simulink model "M_DYN"  (R2022a)
settings: Solver=ode4  StartTime=0.0  StopTime=0.04  FixedStep=0.01  RelTol=1e-3
PreLoadFcn:
  | listing = dir;
  | if (contains([listing .name], 'FLCC')) && (contains([listing .name], 'DYN'))
  |     addpath('./DYN', './FLCC');
  | elseif (contains([listing .name], 'M_DYN.slx'))
  |     addpath('../DYN', '../FLCC');
  | else
  | 
  | end
  | 
  | load('f16data.mat');
  | load('BUS_STRUCTURE_DYN.mat');
  | load('BUS_STRUCTURE_FLCC.mat');
InitFcn:
  | listing = dir;
  | if (contains([listing .name], 'FLCC')) && (contains([listing .name], 'DYN'))
  |     addpath('./DYN', './FLCC');
  | elseif (contains([listing .name], 'M_DYN.slx'))
  |     addpath('../DYN', '../FLCC');
  | else
  | 
  | end
  | 
  | load('f16data.mat');
  | load('BUS_STRUCTURE_DYN.mat');
  | load('BUS_STRUCTURE_FLCC.mat');
values from neighbouring files (symbols this model uses):
  f16data =     [f16data.mat]
libraries: simulink_extras x6, aerolibatmos2 x1
settings Model: Creator=ASCL  LastModifiedBy=ASCL
settings DataIOCC: SaveOutput=off  SignalLogging=off  DSMLogging=off  SaveTime=off  ReturnWorkspaceOutputs=off
settings OptimizationCC: BlockReduction=off  DefaultParameterBehavior=Inlined  UseDivisionForNetSlopeComputation=on  GainParamInheritBuiltInType=on  UseFloatMulNetSlope=on  ExpressionFolding=off  PassReuseOutputArgsAs=Individual arguments  ZeroExternalMemoryAtStartup=off  ZeroInternalMemoryAtStartup=off  EfficientFloat2IntCast=on  LifeSpan=inf  OptimizeBlockOrder=speed  DifferentSizesBufferReuse=on  EfficientTunableParamExpr=on
settings DebuggingCC: SignalInfNanChecking=warning  ReadBeforeWriteMsg=EnableAllAsError  WriteAfterWriteMsg=EnableAllAsError  WriteAfterReadMsg=EnableAllAsError  IntegerOverflowMsg=error  ParameterTunabilityLossMsg=error  UniqueDataStoreMsg=error  AssertControl=DisableAll  NonBusSignalsTreatedAsBus=error  SFInvalidInputDataAccessInChartInitDiag=error  SFTransitionOutsideNaturalParentDiag=error  SFUnreachableExecutionPathDiag=error  SFUndirectedBroadcastEventsDiag=error  IntegerSaturationMsg=error
settings HardwareCC: ProdBitPerPointer=32  ProdBitPerSizeT=32  ProdBitPerPtrDiffT=32  ProdLargestAtomicInteger=Long  ProdLargestAtomicFloat=Double  ProdEndianess=BigEndian  ProdWordSize=32  ProdLongLongMode=on  ProdHWDeviceType=Freescale->MPC83xx
settings ModelReferenceCC: ModelReferenceNumInstancesAllowed=Single
settings SFSimCC: CompileTimeRecursionLimit=0  EnableRuntimeRecursion=off  MATLABDynamicMemAlloc=off
settings RTWCC: SystemTargetFile=ert.tlc  TemplateMakefile=ert_default_tmf  GenerateReport=on  RTWUseSimCustomCode=on  BuildConfiguration=Faster Runs  IncludeHyperlinkInReport=on  LaunchReport=on  GenerateTraceInfo=on  GenerateTraceReport=on  GenerateTraceReportSl=on  GenerateTraceReportSf=on  GenerateTraceReportEml=on
settings CodeAppCC: ForceParamTrailComments=on  IgnoreCustomStorageClasses=off  OperatorAnnotations=on  SimulinkDataObjDesc=on  SFDataObjDesc=on  MATLABFcnDesc=on  InsertBlockDesc=on  StateflowObjectComments=on  MATLABSourceComments=on  EnableCustomComments=on  InlinedPrmAccess=Macros  ReqsInCode=on
settings ERTTargetCC: TargetLangStandard=C99 (ISO)  UtilityFuncGeneration=Shared location  GenerateSampleERTMain=on  IncludeMdlTerminateFcn=off  CombineSignalStateStructs=on  SupportAbsoluteTime=off  SupportNonFinite=off  SupportVariableSizeSignals=on  ParenthesesLevel=Standards  CastingMode=Standards  GenerateSharedConstants=off  InlinedParameterPlacement=NonHierarchical  ERTCustomFileTemplate=example_file_process.tlc  RateTransitionBlockCode=Function  PreserveIfCondition=on  ConvertIfToSwitch=off  EnableSignedLeftShifts=off  EnableSignedRightShifts=off

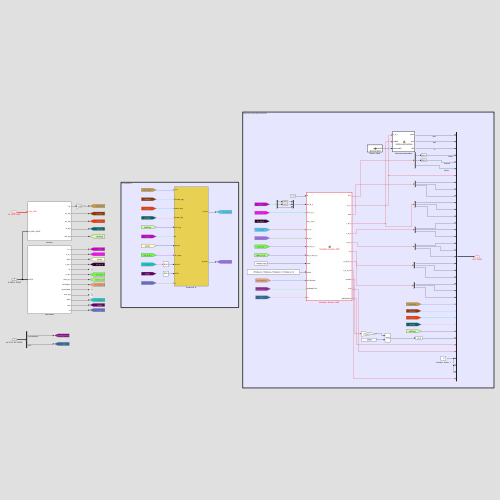
[thumbnail: Simulink's stored preview of the top-level diagram]
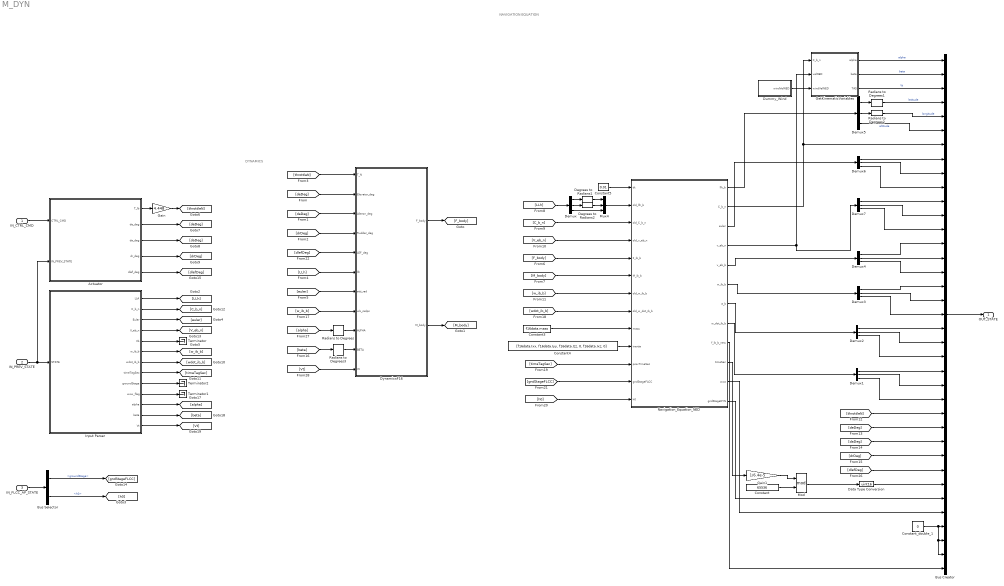
== system M_DYN ==
  note: DYNAMICS
  note: NAVIGATION EQUATION
  IN_CTRL_CMD : Inport  OutDataTypeStr=Bus: BUS_FLCC_CTRL_CMD  Interpolate=off  BusOutputAsStruct=on
  IN_PREV_STATE : Inport  Port=2  OutDataTypeStr=Bus: BUS_DYN_STATE  Interpolate=off  BusOutputAsStruct=on
  IN_FLCC_AP_STATE : Inport  Port=3  OutDataTypeStr=Bus: BUS_FLCC_AP_STATE  BusOutputAsStruct=on
  Actuator : Subsystem
  Bus Creator : BusCreator  Inputs=37  OutDataTypeStr=Bus: BUS_DYN_STATE  NonVirtualBus=on
      settings: InheritFromInputs=off
  Bus Selector : BusSelector  OutputSignals=groundStage,h0
  Constant : Constant  Value=65536
  Constant3 : Constant  Value=f16data.mass
  Constant4 : Constant  Value=[f16data.Ixx, f16data.Iyy, f16data.Izz, 0, f16data.Ixz, 0]
  Constant5 : Constant  Value=0.01
  Constant_double_1 : Constant  Value=0  OutDataTypeStr=double
  Data Type Conversion : DataTypeConversion  OutDataTypeStr=uint16  RndMeth=Round  SaturateOnIntegerOverflow=off
  Degrees to Radians1 : simulink_extras/Transformations/Degrees to Radians
  Degrees to Radians2 : simulink_extras/Transformations/Degrees to Radians
  Demux{,1..7} (8 alike) : Demux  Outputs=3
  Dummy_Wind : MATLAB Function  TreatAsAtomicUnit=on
  DynamicsF16 : Subsystem
  Gain : Gain  Gain=4.448
  Gain1 : Gain  Gain=1/6.4e-5
  GetKinematicVariables : MATLAB Function  TreatAsAtomicUnit=on
  Input Parser : Subsystem
  Mod : Math  Operator=mod  OutputSignalType=real
  Mux4 : Mux  Inputs=3
  Navigation_Equation_NED : MATLAB Function  TreatAsAtomicUnit=on
  Radians to Degrees{,1..3} (4 alike) : simulink_extras/Transformations/Radians to Degrees
  Terminator : Terminator
  Terminator1 : Terminator
  Terminator2 : Terminator
  OUT_STATE : Outport  OutDataTypeStr=Bus: BUS_DYN_STATE  VectorParamsAs1DForOutWhenUnconnected=off  BusOutputAsStruct=on
  wires:
  Actuator/4(dr_deg) -> [drDeg]
  Demux/2 -> Degrees to Radians2/1
  Demux6/3 -> Bus Creator/10
  Navigation_Equation_NED/2(C_b_n) -> Bus Creator/7, GetKinematicVariables/1(C_b_n)
  Navigation_Equation_NED/10(timeSec) -> Gain1/1
  Data Type Conversion/1 -> Bus Creator/31
  [deDeg] -> DynamicsF16/2(Elevator_deg)
  Navigation_Equation_NED/3(euler) -> Demux6/1
  [timeTagSec] -> Navigation_Equation_NED/11(prevTimeSec)
  Demux1/3 -> Bus Creator/25
  Demux1/2 -> Bus Creator/24
  [F_body] -> Navigation_Equation_NED/5(F_ib_b)
  Demux6/1 -> Bus Creator/8
  Demux3/3 -> Bus Creator/19
  Navigation_Equation_NED/7(a_b) -> Demux2/1
  Demux/3 -> Mux4/3
  Navigation_Equation_NED/5(v_eb_b) -> Demux4/1
  Mux4/1 -> Navigation_Equation_NED/2(old_llh_b)
  Demux3/1 -> Bus Creator/17
  [C_b_n] -> Navigation_Equation_NED/3(old_C_b_n)
  Demux4/2 -> Bus Creator/15
  [w_ib_b] -> DynamicsF16/8(wb_radps)
  [drDeg] -> DynamicsF16/4(Rudder_deg)
  Demux1/1 -> Bus Creator/23
  [euler] -> DynamicsF16/7(atti_rad)
  Demux4/3 -> Bus Creator/16
  [daDeg] -> Bus Creator/28
  Demux3/2 -> Bus Creator/18
  Degrees to Radians2/1 -> Mux4/2
  [wdot_ib_b] -> Navigation_Equation_NED/8(old_w_dot_ib_b)
  Actuator/1(T_lb) -> Gain/1
  Input Parser/3(Euler) -> [euler]
  Actuator/3(da_deg) -> [daDeg]
  Radians to Degrees2/1 -> Bus Creator/5  "longitude"
  Demux4/1 -> Bus Creator/14
  Input Parser/1(LLA) -> [LLh]
  IN_CTRL_CMD/1 -> Actuator/1(CTRL_CMD)
  Actuator/2(de_deg) -> [deDeg]
  [daDeg] -> DynamicsF16/3(Aileron_deg)
  Demux6/2 -> Bus Creator/9
  [V_eb_n] -> Navigation_Equation_NED/4(old_v_eb_n)
  [deDeg] -> Bus Creator/27
  Navigation_Equation_NED/1(llh_b) -> Demux5/1
  Demux2/2 -> Bus Creator/21
  Degrees to Radians1/1 -> Mux4/1
  Input Parser/6(w_ib_b) -> [w_ib_b]
  Demux2/3 -> Bus Creator/22
  DynamicsF16/1(F_body) -> [F_body]
  Constant5/1 -> Navigation_Equation_NED/1(dt)
  Bus Creator/1 -> OUT_STATE/1
  Demux5/2 -> Radians to Degrees2/1
  [w_ib_b] -> Navigation_Equation_NED/7(old_w_ib_b)
  Input Parser/7(wdot_ib_b) -> [wdot_ib_b]
  Input Parser/8(timeTagSec) -> [timeTagSec]
  Navigation_Equation_NED/8(w_dot_ib_b) -> Demux1/1
  [LLh] -> DynamicsF16/6(llh)
  Radians to Degrees1/1 -> Bus Creator/4  "latitude"
  [throttleN] -> DynamicsF16/1(T_N)
  Demux5/1 -> Radians to Degrees1/1
  Demux5/3 -> Bus Creator/6  "altitude"
  Gain/1 -> [throttleN]
  [LLh] -> Demux/1
  Demux/1 -> Degrees to Radians1/1
  DynamicsF16/2(M_body) -> [M_body]
  Navigation_Equation_NED/4(v_eb_n) -> Demux7/1, GetKinematicVariables/2(velNED)
  Constant4/1 -> Navigation_Equation_NED/10(inertia)
  Constant3/1 -> Navigation_Equation_NED/9(mass)
  [drDeg] -> Bus Creator/29
  Demux2/1 -> Bus Creator/20
  [throttleN] -> Bus Creator/26
  IN_PREV_STATE/1 -> Actuator/2(IN_PREV_STATE), Input Parser/1(STATE)
  [M_body] -> Navigation_Equation_NED/6(M_ib_b)
  Gain1/1 -> Mod/1
  Mod/1 -> Data Type Conversion/1
  Constant/1 -> Mod/2
  Demux7/2 -> Bus Creator/12
  Demux7/1 -> Bus Creator/11
  Demux7/3 -> Bus Creator/13
  Input Parser/4(V_eb_n) -> [V_eb_n]
  Input Parser/2(C_b_n) -> [C_b_n]
  Input Parser/9(groundStage) -> Terminator2/1
  [gndStageFLCC] -> Navigation_Equation_NED/12(gndStageFLCC)
  Navigation_Equation_NED/11(wow) -> Bus Creator/33
  Actuator/5(dlef_deg) -> [dlefDeg]
  [dlefDeg] -> DynamicsF16/5(LEF_deg)
  Dummy_Wind/1(windVelNED) -> GetKinematicVariables/3(windVelNED)
  GetKinematicVariables/1(alpha) -> Bus Creator/1  "alpha"
  GetKinematicVariables/2(beta) -> Bus Creator/2  "beta"
  GetKinematicVariables/3(TAS) -> Bus Creator/3  "Vt"
  [dlefDeg] -> Bus Creator/30
  Constant_double_1/1 -> Bus Creator/34, Bus Creator/36, Bus Creator/35
  Input Parser/11(alpha) -> [alpha]
  Input Parser/12(beta) -> [beta]
  Input Parser/13(Vt) -> [Vt]
  [alpha] -> Radians to Degrees/1
  [beta] -> Radians to Degrees3/1
  [Vt] -> DynamicsF16/11(Vt)
  Radians to Degrees/1 -> DynamicsF16/9(ALPHA)
  Radians to Degrees3/1 -> DynamicsF16/10(BETA)
  Navigation_Equation_NED/12(gndStageDYN) -> Bus Creator/32
  Navigation_Equation_NED/6(w_ib_b) -> Demux3/1
  Navigation_Equation_NED/9(f_ib_b_new) -> Bus Creator/37
  Input Parser/5(Vb) -> Terminator/1
  Input Parser/10(wow_flag) -> Terminator1/1
  IN_FLCC_AP_STATE/1 -> Bus Selector/1
  Bus Selector/1 -> [gndStageFLCC]  "<groundStage>"
  Bus Selector/2 -> [h0]  "<h0>"
  [h0] -> Navigation_Equation_NED/13(h0)

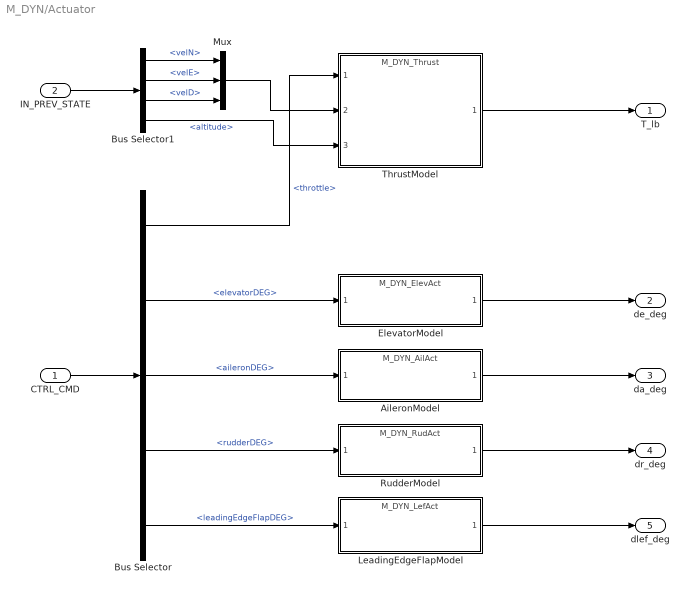
== system M_DYN/Actuator ==
  CTRL_CMD : Inport  OutDataTypeStr=Bus: BUS_FLCC_CTRL_CMD  BusOutputAsStruct=on
  IN_PREV_STATE : Inport  Port=2
  AileronModel : ModelReference  ModelNameDialog=M_DYN_AilAct.slx  ModelReferenceVersion=1.69
  Bus Selector : BusSelector  OutputSignals=throttle,elevatorDEG,aileronDEG,rudderDEG,leadingEdgeFlapDEG
  Bus Selector1 : BusSelector  OutputSignals=velN,velE,velD,altitude
  ElevatorModel : ModelReference  ModelNameDialog=M_DYN_ElevAct.slx  ModelReferenceVersion=1.68
  LeadingEdgeFlapModel : ModelReference  ModelNameDialog=M_DYN_LefAct.slx  SimulationMode=Normal  ModelReferenceVersion=1.75
  Mux : Mux  Inputs=3
  RudderModel : ModelReference  ModelNameDialog=M_DYN_RudAct.slx  ModelReferenceVersion=1.70
  ThrustModel : ModelReference  ModelNameDialog=M_DYN_Thrust.slx  ModelReferenceVersion=1.128
  T_lb : Outport
  de_deg : Outport  Port=2
  da_deg : Outport  Port=3
  dr_deg : Outport  Port=4
  dlef_deg : Outport  Port=5
  wires:
  Bus Selector/1 -> ThrustModel/1  "<throttle>"
  Bus Selector/3 -> AileronModel/1  "<aileronDEG>"
  Bus Selector/2 -> ElevatorModel/1  "<elevatorDEG>"
  Bus Selector/4 -> RudderModel/1  "<rudderDEG>"
  CTRL_CMD/1 -> Bus Selector/1
  ThrustModel/1 -> T_lb/1
  ElevatorModel/1 -> de_deg/1
  RudderModel/1 -> dr_deg/1
  AileronModel/1 -> da_deg/1
  IN_PREV_STATE/1 -> Bus Selector1/1
  Bus Selector1/1 -> Mux/1  "<velN>"
  Bus Selector1/2 -> Mux/2  "<velE>"
  Bus Selector1/3 -> Mux/3  "<velD>"
  Bus Selector1/4 -> ThrustModel/3  "<altitude>"
  Mux/1 -> ThrustModel/2
  LeadingEdgeFlapModel/1 -> dlef_deg/1
  Bus Selector/5 -> LeadingEdgeFlapModel/1  "<leadingEdgeFlapDEG>"

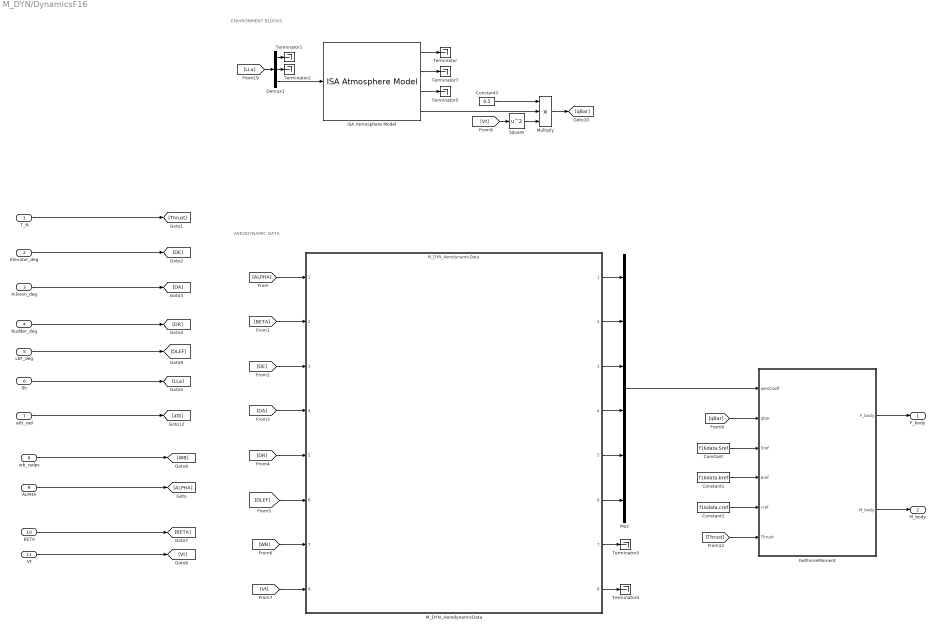
== system M_DYN/DynamicsF16 ==
  note: AERODYNAMIC DATA
  note: ENVIRONMENT BLOCKS
  T_N : Inport
  Elevator_deg : Inport  Port=2
  Aileron_deg : Inport  Port=3
  Rudder_deg : Inport  Port=4
  LEF_deg : Inport  Port=5
  llh : Inport  Port=6
  atti_rad : Inport  Port=7
  wb_radps : Inport  Port=8
  ALPHA : Inport  Port=9
  BETA : Inport  Port=10
  Vt : Inport  Port=11
  Constant : Constant  Value=f16data.Sref
  Constant1 : Constant  Value=f16data.bref
  Constant2 : Constant  Value=f16data.cref
  Constant3 : Constant  Value=0.5
  Demux1 : Demux  Outputs=3
  GetForceMoment : MATLAB Function  TreatAsAtomicUnit=on
  ISA Atmosphere Model : aerolibatmos2/ISA Atmosphere Model  custom=off  g=9.80665  gamma=1.4  R=287.0531  L=0.0065  h_trop=11000  h_strat=20000  rho0=1.225  P0=101325  T0=288.15  h0=0
  M_DYN_AerodynamicData : ModelReference  ModelNameDialog=M_DYN_AerodynamicData.slx  SimulationMode=Normal  ModelReferenceVersion=1.96
  Multiply : Product  Inputs=3
  Mux : Mux  Inputs=6
  Square : Math  Operator=square  SignedPower=on
  Terminator{,1..5,7} (7 alike) : Terminator
  F_body : Outport  VectorParamsAs1DForOutWhenUnconnected=off
  M_body : Outport  Port=2  VectorParamsAs1DForOutWhenUnconnected=off
  wires:
  ISA Atmosphere Model/4 -> Multiply/2
  ISA Atmosphere Model/1 -> Terminator/1
  ISA Atmosphere Model/3 -> Terminator5/1
  T_N/1 -> [Thrust]
  Elevator_deg/1 -> [DE]
  Aileron_deg/1 -> [DA]
  Rudder_deg/1 -> [DR]
  atti_rad/1 -> [atti]
  llh/1 -> [LLa]
  [LLa] -> Demux1/1
  Demux1/3 -> ISA Atmosphere Model/1
  Demux1/1 -> Terminator1/1
  Demux1/2 -> Terminator2/1
  LEF_deg/1 -> [DLEF]
  [ALPHA] -> M_DYN_AerodynamicData/1
  [BETA] -> M_DYN_AerodynamicData/2
  [DE] -> M_DYN_AerodynamicData/3
  [DA] -> M_DYN_AerodynamicData/4
  [DR] -> M_DYN_AerodynamicData/5
  [DLEF] -> M_DYN_AerodynamicData/6
  [WB] -> M_DYN_AerodynamicData/7
  wb_radps/1 -> [WB]
  [Vt] -> M_DYN_AerodynamicData/8
  M_DYN_AerodynamicData/1 -> Mux/1
  M_DYN_AerodynamicData/2 -> Mux/2
  M_DYN_AerodynamicData/3 -> Mux/3
  M_DYN_AerodynamicData/4 -> Mux/4
  M_DYN_AerodynamicData/5 -> Mux/5
  M_DYN_AerodynamicData/6 -> Mux/6
  Mux/1 -> GetForceMoment/1(aeroCoeff)
  GetForceMoment/1(F_body) -> F_body/1
  GetForceMoment/2(M_body) -> M_body/1
  [qBar] -> GetForceMoment/2(qbar)
  Constant/1 -> GetForceMoment/3(Sref)
  Constant2/1 -> GetForceMoment/5(cref)
  Constant1/1 -> GetForceMoment/4(bref)
  [Thrust] -> GetForceMoment/6(Thrust)
  ISA Atmosphere Model/2 -> Terminator7/1
  [Vt] -> Square/1
  Square/1 -> Multiply/3
  Constant3/1 -> Multiply/1
  Multiply/1 -> [qBar]
  M_DYN_AerodynamicData/8 -> Terminator4/1
  M_DYN_AerodynamicData/7 -> Terminator3/1
  ALPHA/1 -> [ALPHA]
  BETA/1 -> [BETA]
  Vt/1 -> [Vt]

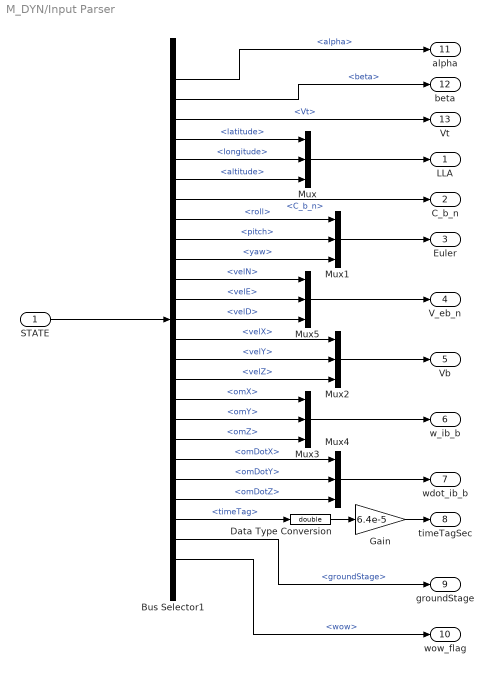
== system M_DYN/Input Parser ==
  STATE : Inport  OutDataTypeStr=Bus: BUS_DYN_STATE
  Bus Selector1 : BusSelector  OutputSignals=alpha,beta,Vt,latitude,longitude,altitude,C_b_n,roll,pitch,yaw,velN,velE,velD,velX,velY,velZ,omX,omY,omZ,omDotX,omDotY,omDotZ,timeTag,groundStage,wow
  Data Type Conversion : DataTypeConversion  OutDataTypeStr=double  SaturateOnIntegerOverflow=off  RndMeth=Floor
  Gain : Gain  Gain=6.4e-5
  Mux{,1..5} (6 alike) : Mux  Inputs=3
  LLA : Outport
  C_b_n : Outport  Port=2
  Euler : Outport  Port=3
  V_eb_n : Outport  Port=4
  Vb : Outport  Port=5
  w_ib_b : Outport  Port=6
  wdot_ib_b : Outport  Port=7
  timeTagSec : Outport  Port=8
  groundStage : Outport  Port=9
  wow_flag : Outport  Port=10
  alpha : Outport  Port=11
  beta : Outport  Port=12
  Vt : Outport  Port=13
  wires:
  Bus Selector1/5 -> Mux/2  "<longitude>"
  Bus Selector1/4 -> Mux/1  "<latitude>"
  Bus Selector1/6 -> Mux/3  "<altitude>"
  Mux3/1 -> w_ib_b/1
  Mux/1 -> LLA/1
  STATE/1 -> Bus Selector1/1
  Bus Selector1/18 -> Mux3/2  "<omY>"
  Bus Selector1/19 -> Mux3/3  "<omZ>"
  Bus Selector1/17 -> Mux3/1  "<omX>"
  Bus Selector1/16 -> Mux2/3  "<velZ>"
  Bus Selector1/15 -> Mux2/2  "<velY>"
  Bus Selector1/14 -> Mux2/1  "<velX>"
  Bus Selector1/10 -> Mux1/3  "<yaw>"
  Bus Selector1/9 -> Mux1/2  "<pitch>"
  Bus Selector1/8 -> Mux1/1  "<roll>"
  Mux1/1 -> Euler/1
  Mux2/1 -> Vb/1
  Bus Selector1/21 -> Mux4/2  "<omDotY>"
  Bus Selector1/20 -> Mux4/1  "<omDotX>"
  Bus Selector1/22 -> Mux4/3  "<omDotZ>"
  Mux4/1 -> wdot_ib_b/1
  Bus Selector1/23 -> Data Type Conversion/1  "<timeTag>"
  Data Type Conversion/1 -> Gain/1
  Gain/1 -> timeTagSec/1
  Bus Selector1/7 -> C_b_n/1  "<C_b_n>"
  Bus Selector1/12 -> Mux5/2  "<velE>"
  Bus Selector1/11 -> Mux5/1  "<velN>"
  Bus Selector1/13 -> Mux5/3  "<velD>"
  Mux5/1 -> V_eb_n/1
  Bus Selector1/24 -> groundStage/1  "<groundStage>"
  Bus Selector1/25 -> wow_flag/1  "<wow>"
  Bus Selector1/1 -> alpha/1  "<alpha>"
  Bus Selector1/2 -> beta/1  "<beta>"
  Bus Selector1/3 -> Vt/1  "<Vt>"

== matlab function M_DYN/Dummy_Wind ==
  data: windVelNED output
function windVelNED = Dummy_Wind()
windVelNED = zeros(3,1);

== matlab function M_DYN/DynamicsF16/GetForceMoment ==
  data: F_body output; M_body output; aeroCoeff input; qbar input; Sref input; bref input; cref input; Thrust input
function [F_body, M_body] = GetForceMoment(aeroCoeff, qbar, Sref, bref, cref, Thrust)

F_body = zeros(3,1);
M_body = zeros(3,1);

% Force [N]
F_body(1) = aeroCoeff(1) * qbar * Sref + Thrust;
F_body(2) = aeroCoeff(2) * qbar * Sref;
F_body(3) = aeroCoeff(3) * qbar * Sref;

% Moment [N-m]
M_body(1) = aeroCoeff(4) * qbar * Sref * bref;
M_body(2) = aeroCoeff(5) * qbar * Sref * cref;
M_body(3) = aeroCoeff(6) * qbar * Sref * bref;

== matlab function M_DYN/Navigation_Equation_NED ==
  data: dt input; llh_b output; old_llh_b input; old_C_b_n input; old_v_eb_n input; F_ib_b input; M_ib_b input; old_w_ib_b input; old_w_dot_ib_b input; mass input; inertia input; C_b_n output; euler output; v_eb_n output; v_eb_b output; w_ib_b output; a_b output; w_dot_ib_b output; f_ib_b_new output; timeSec output; prevTimeSec input; gndStageFLCC input; wow output; h0 input; gndStageDYN output
function [llh_b, C_b_n, euler, v_eb_n, v_eb_b, w_ib_b, a_b, w_dot_ib_b, f_ib_b_new, timeSec, wow, gndStageDYN]   = Navigation_Equation_NED(dt, old_llh_b, old_C_b_n, old_v_eb_n, F_ib_b, M_ib_b, old_w_ib_b, old_w_dot_ib_b, mass, inertia, prevTimeSec, gndStageFLCC, h0)
% Reference:    Groves, Paul D. "Principles of GNSS, inertial, and 
%               multisensor integrated navigation systems, [Book review]."
%               IEEE Aerospace and Electronic Systems Magazine 30.2 (2015): 26-27.
%
% INPUTS:
%   dt          time interval between updates [s]
%   old_llh_b   previous latitude, longitude, height [rad, rad, m]
%   old_C_b_n   previous body-to-NED coordinate transformation matrix
%   old_v_eb_n  previous velocity of body frame w.r.t. ECEF frame,
%               resolved along north, east, and down [m/s]
%   F_ib_b      (non-gravitational) force of body frame w.r.t.
%               ECEF frame, resolved along body-frame axes, averaged over
%               time interval [m/s^2]
%   M_ib_b      net moment of body frame w.r.t. ECI frame, 
%               resolved about body-frame axes [kg m^2 rad/s]
%   old_w_ib_b  previous body angular rate w.r.t. ECI frame,
%               resolved about body axes [rad/s]
%   old_w_dot_ib_b
%               previous time rate of body angular rate w.r.t. ECI frame,
%               resolved about body axes [rad/s^2]
%   mass        [kg]
%   inertia     [kg m^2]
%   prevTimeSec [sec]
%   prevFlightStage uint8 flag
%
% OUTPUTS: 
%   llh_b       latitude, longitude, height [rad, rad, m]
%   C_b_n       body-to-NED coordinate transformation matrix
%   v_eb_n      velocity of body frame w.r.t. ECEF frame,
%               resolved along north, east, and down [m/s]
%   w_ib_b      body angular rate [rad/s]
%   w_dot_ib_b  time rate of body angular rate [rad/s^2]
%   a_b         body acceleration [m/s^2]
%   euler       [rad]
%   v_eb_b      body velocity [m/s]
%   timeSec     [sec]
%   flightStage uint8
%   wow         boolean

%% [0] Initialize Outputs
llh_b   = zeros(3,1);
C_b_n   = zeros(3,3);
v_eb_n  = zeros(3,1);
w_ib_b  = zeros(3,1);
w_dot_ib_b  = zeros(3,1);
a_b     = zeros(3,1);
euler   = zeros(3,1);
v_eb_b  = zeros(3,1);
f_ib_b_new = zeros(3,1);
timeSec = 0;
wow = true;
gndStageDYN = gndStageFLCC;

if gndStageDYN == uint8(9)
    llh_b = old_llh_b;
    timeSec = prevTimeSec + dt;
    return
else
end

%% [1] Define Constant Parameters
w_ie    = 7.2921159E-5;     % Earth rotation rate [rad/s]
R_0     = 6378137;          % WGS84 Equatorial radius [m]
R_P     = 6356752.31425;    %WGS84 Polar radius [m]
e       = 0.0818191908425;  % WGS84 eccentricity
f       = 1 / 298.257223563;%WGS84 flattening
mu      = 3.986004418E14;   %WGS84 Earth gravitational constant [m^3 s^-2]

Ib      = [inertia(1), -inertia(4), -inertia(5);...
          -inertia(4),  inertia(2), -inertia(6);...
          -inertia(5), -inertia(6),  inertia(3)];
%                           % Moment of inertia [kg m^2]

% Tolerance for compared to zero operation
TOL     = eps(0.5);

%% [2] ATTITUDE UPDATE

% Calculate w_ib_b: angular rate of body frame w.r.t. ECI frame,
%           resolved about body axes, averaged over time interval [rad/s]
w_dot_ib_b  = Ib\(M_ib_b - cross(old_w_ib_b, Ib*old_w_ib_b));
% w_ib_b      = old_w_ib_b + 0.5 * dt * (w_dot_ib_b + old_w_dot_ib_b); 
w_ib_b      = old_w_ib_b + dt * w_dot_ib_b;

% START: TRICK for ground motion ------------------------------------------
if gndStageDYN <= uint8(4)
    w_ib_b(1) = 0.0;
    w_ib_b(2) = 0.0;
    w_dot_ib_b = (w_ib_b - old_w_ib_b ) / (0.5*dt) - old_w_dot_ib_b;
end
% END: TRICK for ground motion --------------------------------------------

% First, Calculate attitude increment, magnitude, and skew-symmetric matrix
alpha_ib_b  = w_ib_b * dt;
if abs(alpha_ib_b' * alpha_ib_b - 0) < TOL % (alpha_ib_b' * alpha_ib_b == 0)
    mag_alpha   = 0.0;
else
    mag_alpha   = sqrt(alpha_ib_b' * alpha_ib_b);
end

Alpha_ib_b  = [             0, -alpha_ib_b(3),  alpha_ib_b(2); ...
                alpha_ib_b(3),              0, -alpha_ib_b(1); ...
               -alpha_ib_b(2),  alpha_ib_b(1),             0];

w_ie_n      = w_ie * [cos(old_llh_b(1)); 0; -sin(old_llh_b(1))];

% From (5.44), determine the angular rate of the NED frame
% w.r.t the ECEF frame, resolved about NED
old_N_E     = R_0 * (1-e^2) / sqrt( 1 - (e * sin(old_llh_b(1)))^2 );
old_M_E_norm1 = 1 - (e * sin(old_llh_b(1)))^2;
if (old_M_E_norm1 > 0.000001)
    old_M_E_norm2 = sqrt(old_M_E_norm1);
    old_M_E_norm3 = old_M_E_norm1 * old_M_E_norm2;
    old_M_E = R_0 / old_M_E_norm3;
else
    old_M_E_norm2 = 0.0;
    old_M_E_norm3 = 0.0;
    old_M_E = R_0 / 0.97;
end

old_w_en_n = [old_v_eb_n(2) / (old_N_E + old_llh_b(3));...
             -old_v_eb_n(1) / (old_M_E + old_llh_b(3));...
             -old_v_eb_n(2) * tan(old_llh_b(1)) / (old_N_E + old_llh_b(3))];


%% [3] SPECIFIC FORCE FRAME TRANSFORMATION
% Calculate ave_C_b_e: the average body-to-ECEF-frame transformation matrix
%           over the update interval using (5.84) and (5.85)
temp_w_enie_n   = old_w_en_n + w_ie_n;
skew_w_enie_n   = [               0,-temp_w_enie_n(3), temp_w_enie_n(2);...
                   temp_w_enie_n(3),                0,-temp_w_enie_n(1);...
                  -temp_w_enie_n(2), temp_w_enie_n(1),                0];

if (mag_alpha > 1.E-8)
    ave_C_b_n = old_C_b_n * (eye(3) + (1 - cos(mag_alpha)) / mag_alpha^2 ...
        * Alpha_ib_b + (1 - sin(mag_alpha) / mag_alpha) / mag_alpha^2 ...
        * Alpha_ib_b * Alpha_ib_b) ...
        - 0.5 * skew_w_enie_n * old_C_b_n;
else
     ave_C_b_n = old_C_b_n ...
        - 0.5 * skew_w_enie_n * old_C_b_n;
end %if mag_alpha     

% Orthonormalize DCM
ave_C_b_n   = quat2rotm(quatnormalize(rotm2quat(ave_C_b_n)));

% Transform specific force to ECEF-frame resolving axes using (5.86)
f_ib_b = F_ib_b / mass;
f_ib_n = ave_C_b_n * f_ib_b;


%% [4] UPDATE VELOCITY
% Calculate acceleration due to gravity resolved about NED
grav_n = zeros(3,1);

% Calculate surface gravity using the Somigliana model, (2.134)
sinsqL = sin(old_llh_b(1))^2;
g_0 = 9.7803253359 * (1 + 0.001931853 * sinsqL) / sqrt(1 - e^2 * sinsqL);

% Calculate north gravity using (2.140)
grav_n(1) = -8.08E-9 * old_llh_b(3) * sin(2 * old_llh_b(1));

% East gravity is zero
grav_n(2) = 0.0;

% Calculate down gravity using (2.139)
grav_n(3) = g_0 ...
    * (1 - (2 / R_0) * (1 + f * (1 - 2 * sinsqL) + (w_ie^2 * R_0^2 * R_P / mu)) ...
    * old_llh_b(3) + (3 * old_llh_b(3)^2 / R_0^2));

% Calculate Skew-symmetric matrix for Coriolis and transport-rate term
w_CnT   = old_w_en_n + 2 * w_ie_n;
skew_w_CnT  = [       0, -w_CnT(3),  w_CnT(2); ...
               w_CnT(3),         0, -w_CnT(1); ...
              -w_CnT(2),  w_CnT(1),         0];

% START: TRICK for ground motion ------------------------------------------
if gndStageDYN <= uint8(4)
    normalA = (-grav_n(3) + skew_w_CnT(3,:) * old_v_eb_n) - f_ib_n(3);

    f_ib_n(3) = -grav_n(3) + skew_w_CnT(3,:) * old_v_eb_n;

    temp = f_ib_n(1) -0.3 * sign(f_ib_n(1)) * abs(normalA);
    if temp * f_ib_n(1) < 0
        f_ib_n(1) = 0.0;
    else
        f_ib_n(1) = temp;
    end
    temp = f_ib_n(2) -0.3 * sign(f_ib_n(2)) * abs(normalA);
    if temp * f_ib_n(2) < 0
        f_ib_n(2) = 0.0;
    else
        f_ib_n(2) = temp;
    end
%     f_ib_n(1) = f_ib_n(1) -0.3 * sign(f_ib_n(1)) * abs(normalA);
%     f_ib_n(2) = f_ib_n(2) -0.3 * sign(f_ib_n(2)) * abs(normalA);
    if gndStageDYN <= uint8(1)
        f_ib_n(1) = 0.0;
        f_ib_n(2) = 0.0;
    end
    f_ib_b = ave_C_b_n' * f_ib_n;
elseif gndStageDYN == uint8(5)
    f_ib_n(3) = max(-99999, min(f_ib_n(3), -grav_n(3) + skew_w_CnT(3,:) * old_v_eb_n));
else
end
f_ib_b_new = f_ib_b;
% END: TRICK for ground motion --------------------------------------------

% From (5.54),
v_eb_n = old_v_eb_n ...
    + dt * f_ib_n ...
    + dt * grav_n ...
    - dt * skew_w_CnT * old_v_eb_n;

% START: TRICK for ground motion ------------------------------------------
if gndStageDYN <= uint8(4)
    v_eb_n(3) = 0.0;
    if gndStageDYN <= uint8(1)
        v_eb_n(1) = 0.0;
        v_eb_n(2) = 0.0;
    end
else
end
% END: TRICK for ground motion --------------------------------------------

%% [5] UPDATE CURVILINEAR POSITION
% Update height using (5.56)
llh_b(3)    = old_llh_b(3) ...
    - dt/2 * (old_v_eb_n(3) + v_eb_n(3));

% Update latitude using (5.56)
llh_b(1)    = old_llh_b(1) ...
    + dt/2 * old_v_eb_n(1) / (old_M_E + old_llh_b(3)) ...
    + dt/2 * v_eb_n(1) / (old_M_E + llh_b(3));

% Calculate meridian and transverse radii of curvature
N_E         = R_0 * (1-e^2) / sqrt( 1 - (e * sin(llh_b(1)))^2 );
M_E_norm1 = 1 - (e * sin(llh_b(1)))^2;
if (M_E_norm1 > 0.000001)
    M_E_norm2 = sqrt(M_E_norm1);
    M_E_norm3 = M_E_norm1 * M_E_norm2;
    M_E = R_0 / M_E_norm3;
else
    M_E_norm2 = 0.0;
    M_E_norm3 = 0.0;
    M_E = R_0 / 0.97;
end
% M_E         = R_0 / ( 1 - (e * sin(llh_b(1)))^2 )^1.5;


% Update longitude using (5.56)
llh_b(2)    = old_llh_b(2) ...
    + dt/2 * old_v_eb_n(2) / ((old_N_E + old_llh_b(3)) * cos(old_llh_b(1))) ...
    + dt/2 * v_eb_n(2) / ((N_E + llh_b(3)) * cos(llh_b(1)));

%% [6] UPDATE ATTITUDE
% From (5.44), determine the angular rate of the NED frame
% w.r.t the ECEF frame, resolved about NED frame
w_en_n  = [v_eb_n(2) / (N_E + llh_b(3));...
          -v_eb_n(1) / (M_E + llh_b(3));...
          -v_eb_n(2) * tan(llh_b(1)) / (N_E + llh_b(3))];                    

% Obtain coordinate transformation matrix from the new attitude w.r.t. an
% inertial frame to the old using Rodrigues' formula, (5.73)
if mag_alpha>1.E-8
    C_new_old = eye(3) + sin(mag_alpha) / mag_alpha * Alpha_ib_b +...
        (1 - cos(mag_alpha)) / mag_alpha^2 * Alpha_ib_b * Alpha_ib_b;
else
    C_new_old = eye(3) + Alpha_ib_b;
end %if mag_alpha    

% Update attitude using (5.77)
ave_w_ie_n  = w_ie_n + 0.5 * w_en_n + 0.5 * old_w_en_n;
skew_w_ie_n = [            0, -ave_w_ie_n(3),  ave_w_ie_n(2); ...
               ave_w_ie_n(3),              0, -ave_w_ie_n(1); ...
              -ave_w_ie_n(2),  ave_w_ie_n(1),              0];

C_b_n   = (eye(3) - skew_w_ie_n * dt) * old_C_b_n * C_new_old;

% Orthonormalize DCM
C_b_n   = quat2rotm(quatnormalize(rotm2quat(C_b_n)));
 

%% [7] CALCULATE EULER ANGLES
C_n_b = C_b_n';

% if abs(C_n_b(1,3)) > 1
%     fprintf("%2.5f, %2.5f, %2.5f \r\n", C_b_n(1,1), C_b_n(1,2), C_b_n(1,3));
%     fprintf("%2.5f, %2.5f, %2.5f \r\n", C_b_n(2,1), C_b_n(2,2), C_b_n(2,3));
%     fprintf("%2.5f, %2.5f, %2.5f \r\n", C_b_n(3,1), C_b_n(3,2), C_b_n(3,3));
% end

% euler(1,1) = atan2(C_n_b(2,3),C_n_b(3,3));  % roll
% euler(2,1) = - asin(C_n_b(1,3));        % pitch
% euler(3,1) = atan2(C_n_b(1,2),C_n_b (1,1));  % yaw

C23 = C_n_b(2,3);
C33 = C_n_b(3,3);

euler(1,1) = atan2(C23, C33);  % roll
if isnan(euler(1,1))
    euler(1,1) = 0.0;
end
euler(2,1) = - asin(C_n_b(1,3));        % pitch
euler(3,1) = atan2(C_n_b(1,2),C_n_b (1,1));  % yaw
if isnan(euler(3,1))
    euler(3,1) = 0.0;
end


%% [8] CALCULATE BODY VELOCITY
% v_eb_b  = C_n_b * v_eb_n;
v_eb_b  = C_n_b * v_eb_n;
% a_b = f_ib_b + ave_C_b_n' * grav_n;
a_b = f_ib_b + C_n_b * grav_n;

% START: TRICK for ground motion ------------------------------------------
if gndStageDYN <= uint8(4)
%     a_n = C_b_n * a_b;
%     a_n(3) = 0.0;
%     a_b = C_n_b * a_n;
else
end
% END: TRICK for ground motion --------------------------------------------


%% [9] UPDATE TIME SEC
timeSec = prevTimeSec + dt;


%% [11] Calculate WOW flags
% [0 = JUST BOOTED UP]
% [1 = GROUND IDLE]
% [2 = TAXING]
% [3 = READY TAKEOFF]
% [4 = GROUND ROLL]
% [5 = ROTATION]
% [6 = TO AIR TRANSITION]
% [7 = CLIMBOUT]
% [8 = IN FLYING]
% [9 = CRASHES, ABNORMAL]
 
if (gndStageDYN >= uint8(6))
    wow = false;
else
    wow = true;
end

if ( (llh_b(3) < (h0 - 5)) && (gndStageDYN >= uint8(8)) )
    wow = true;
    gndStageDYN = uint8(9);
else

end

== matlab function M_DYN/GetKinematicVariables ==
  data: C_b_n input; alpha output; beta output; TAS output; velNED input; windVelNED input
function [alpha, beta, TAS] = GetKinematicVariables(C_b_n, velNED, windVelNED)
%GetKinematicVariables

% Initialize
alpha   = 0.0;
beta    = 0.0;
TAS     = 0.0;

% Body to NED
% cRol = cos(attiEuler(1));
% sRol = sin(attiEuler(1));
% cPit = cos(attiEuler(2));
% sPit = sin(attiEuler(2));
% cYaw = cos(attiEuler(3));
% sYaw = sin(attiEuler(3));

% Coordinate Transformation
% NED to Body
C_n_b = C_b_n';
% C_n_b   = [              cPit*cYaw,                cPit*sYaw,     -sPit;...
%           sRol*sPit*cYaw-cRol*sYaw, sRol*sPit*sYaw+cRol*cYaw, sRol*cPit;...
%           cRol*sPit*cYaw+sRol*sYaw, cRol*sPit*sYaw-sRol*cYaw, cRol*cPit];

% Velocity relative to the wind
vRA_n = [velNED(1) - windVelNED(1); ...
    velNED(2) - windVelNED(2); ...
    velNED(3) - windVelNED(3)];
vRA_b = C_n_b * vRA_n;

TAS = norm(vRA_n);

% AOA
if (norm(vRA_b) < 0.5)
    alpha = 0.0;
else
    alpha = atan2(vRA_b(3), vRA_b(1));
end

% Sideslip Angle
if ( (abs(vRA_b(2)) < TAS) && (TAS > 0.5) )
    beta    = asin(vRA_b(2) / TAS);
else
    % Abnormal case
    beta    = 0.0;
end
